simulink model "uniaxial_table"  (R2023b)
settings: Solver=ode8  StartTime=0.0  StopTime=30  FixedStep=t_step  MaxStep=1e-6  RelTol=1e-6
values from neighbouring files (symbols this model uses):
  A = 0.012456    [Compute_TFs_and_StateSpace.m]    (also in parameters.m)
  C_l = k_c    (= 8.37005e-08)    [parameters.m]
  c_sp = qsi_sp*2*m_sp*2*pi*f_sp    (= 2513.27412287)    [parameters.m]
  c_t = 5.7800    (= 5.78)    [parameters.m]
  k_c = k_pl/2    (= 8.37005e-08)    [parameters.m]
  K_h = 4*beta_e*A^2/V_t    (= 45213.1716837)    [parameters.m]
  k_p = 1.2993/1e-2    (= 129.93)    [Copy_of_PID_surf_Zeta.m]    (also in PID_surface.m; parameters.m = 1.2993)
  k_q = 1934.50    (= 1934.5)    [parameters.m]
  k_sp = m_sp*(2*pi*f_sp)^2    (= 315827.340835)    [parameters.m]
  k_sv = 1934.50    (= 1934.5)    [parameters.m]
  m_sp = 2000    [parameters.m]
  m_T = m_p    (= 1.9751)    [parameters.m]
  tau_sv = 0.0246    [Compute_TFs_and_StateSpace.m]    (also in parameters.m)
libraries: slpidlib x1
settings Model: Creator=afons  LastModifiedBy=afons

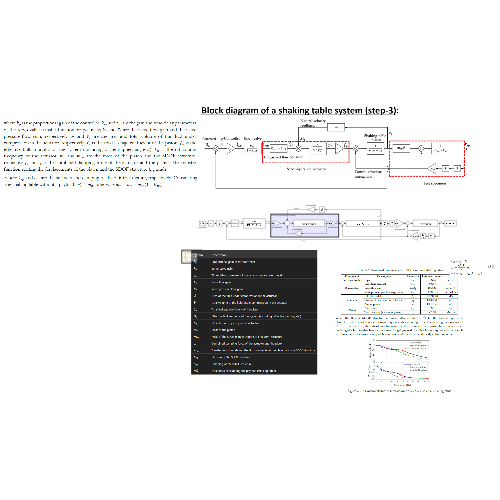
[thumbnail: Simulink's stored preview of the top-level diagram]
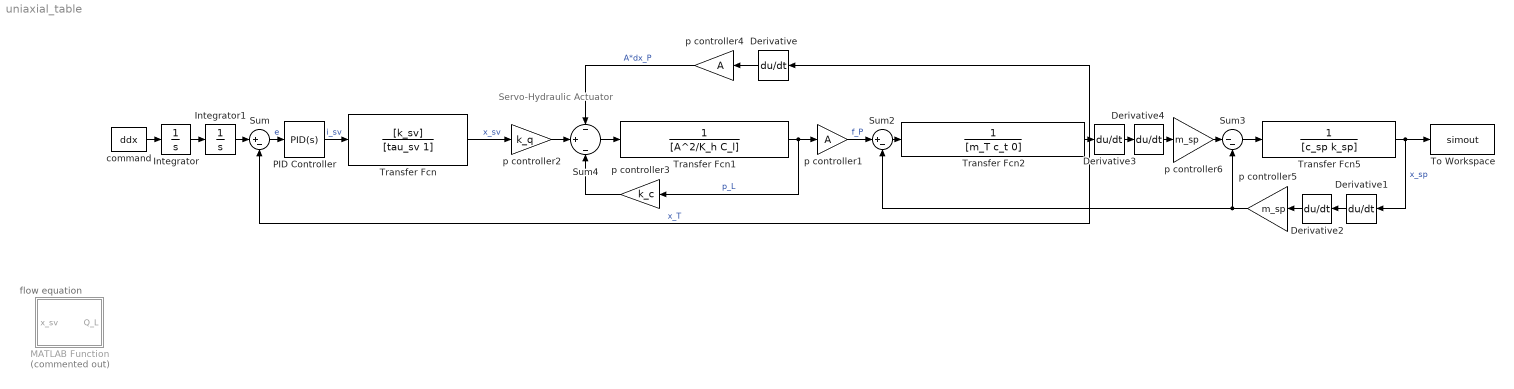
== system uniaxial_table ==
  note: Servo-Hydraulic Actuator
  note: flow equation
  Derivative{,1..4} (5 alike) : Derivative
  Integrator : Integrator
  Integrator1 : Integrator
  MATLAB Function : MATLAB Function  Commented=on  TreatAsAtomicUnit=on
  PID Controller : slpidlib/PID Controller  Controller=PID  Form=Parallel  TimeDomain=Continuous-time  UseExternalTs=off  SampleTime=-1  IntegratorMethod=Forward Euler  FilterMethod=Forward Euler  ControllerParametersSource=internal  P=k_p  I=0  UseKiTs=off  D=0  N=1  UseFilter=on  TunerSelectOption=Transfer Function Based (PID Tuner App)  InitialConditionSource=internal  InitialConditionForIntegrator=0  InitialConditionForFilter=0  DifferentiatorICPrevScaledInput=0  ExternalReset=none  TrackingMode=off  Kt=1  LimitOutput=off  SatLimitsSource=internal  UpperSaturationLimit=inf  LowerSaturationLimit=-inf  LinearizeAsGain=on  AntiWindupMode=none  Kb=1  LimitIntegrator=off  UpperIntegratorSaturationLimit=inf  LowerIntegratorSaturationLimit=-inf  POutMin=[]  POutMax=[]  IOutMin=[]  IOutMax=[]  DOutMin=[]  DOutMax=[]  NOutMin=[]  NOutMax=[]  SumOutMin=[]  SumOutMax=[]  SaturationOutMin=[]  SaturationOutMax=[]  PParamMin=[]  PParamMax=[]  IParamMin=[]  IParamMax=[]  DParamMin=[]  DParamMax=[]  NParamMin=[]  NParamMax=[]  KbParamMin=[]  KbParamMax=[]  KtParamMin=[]  KtParamMax=[]  KbOutMin=[]  KbOutMax=[]  KtOutMin=[]  KtOutMax=[]  IntegratorOutMin=[]  IntegratorOutMax=[]  FilterOutMin=[]  FilterOutMax=[]  SumI1OutMin=[]  SumI1OutMax=[]  SumI2OutMin=[]  SumI2OutMax=[]  SumI3OutMin=[]  SumI3OutMax=[]  SumI4OutMin=[]  SumI4OutMax=[]  SumDOutMin=[]  SumDOutMax=[]  DifferentiatorOutMin=[]  DifferentiatorOutMax=[]  FilterDiffOutCoefMin=[]  FilterDiffOutCoefMax=[]  ReciprocalOutMin=[]  ReciprocalOutMax=[]  SumDenOutMin=[]  SumDenOutMax=[]  SumNumOutMin=[]  SumNumOutMax=[]  DivideOutMin=[]  DivideOutMax=[]  UdiffTsProdOutMin=[]  UdiffTsProdOutMax=[]  NTsProdOutMin=[]  NTsProdOutMax=[]  UintegralTsProdOutMin=[]  UintegralTsProdOutMax=[]  UngainTsProdOutMin=[]  UngainTsProdOutMax=[]  ClampingZeroOutDataTypeStr=Inherit: Inherit via back propagation  ClampingZeroOutMin=[]  ClampingZeroOutMax=[]  FilterDenConstantOutDataTypeStr=Inherit: Inherit via back propagation  FilterDenConstantOutMin=[]  FilterDenConstantOutMax=[]  PCopyOutDataTypeStr=Inherit: Inherit via back propagation  PCopyOutMin=[]  PCopyOutMax=[]  NCopyOutDataTypeStr=Inherit: Inherit via back propagation  NCopyOutMin=[]  NCopyOutMax=[]  IntegratorContinuousStateAttributes=''  IntegratorStateMustResolveToSignalObject=off  IntegratorRTWStateStorageClass=Auto  FilterContinuousStateAttributes=''  FilterStateMustResolveToSignalObject=off  FilterRTWStateStorageClass=Auto  ParallelPVariant=InternalParameters  IdealPVariant=Disabled  IVariant=InternalParameters  DVariant=InternalParameters  IntegratorVariant=Continuous  SatVariant=Disabled  AWVariant=Passthrough  PCopyVariant=Disabled  TRVariant=Disabled  FdbkBlocksVariant=Forward  IdealPFdbkVariant=Disabled  SatFdbkVariant=Disabled  DerivativeFilterVariant=ContFilter  NVariant=InternalParameters  NCopyVariant=Disabled  FilterICVariant=InternalICsFilter  IntegratorICVariant=InternalICs  ExternalResetVariant=Disabled  TRSumVariant=Passthrough  SumFdbkVariant=Disabled  SumVariant=Sum_PID  TsampFilterVariant=InternalTs  TsampNgainVariant=Passthrough  TsampIntegralVariant=Disabled_SignalSpec  ExternalSaturationOutDataTypeStr=Inherit: Same as second input
  Sum : Sum  Inputs=|+-
  Sum2 : Sum  Inputs=|+-
  Sum3 : Sum  Inputs=|--
  Sum4 : Sum  Inputs=-|+|-
  To Workspace : ToWorkspace  VariableName=simout  SaveFormat=Timeseries  SampleTime=-1
  Transfer Fcn : TransferFcn  Numerator=[k_sv]  Denominator=[tau_sv 1]
  Transfer Fcn1 : TransferFcn  Denominator=[A^2/K_h C_l]
  Transfer Fcn2 : TransferFcn  Denominator=[m_T c_t 0]
  Transfer Fcn5 : TransferFcn  Denominator=[c_sp k_sp]
  command : FromWorkspace  VariableName=ddx
  p controller1 : Gain  Gain=A
  p controller2 : Gain  Gain=k_q
  p controller3 : Gain  Gain=k_c
  p controller4 : Gain  Gain=A
  p controller5 : Gain  Gain=m_sp
  p controller6 : Gain  Gain=m_sp
  wires:
  Sum/1 -> PID Controller/1  "e"
  PID Controller/1 -> Transfer Fcn/1  "i_sv"
  Transfer Fcn/1 -> p controller2/1  "x_sv"
  Sum4/1 -> Transfer Fcn1/1
  p controller4/1 -> Sum4/1  "A*dx_P"
  Transfer Fcn1/1 -> p controller1/1, p controller3/1  "p_L"
  p controller1/1 -> Sum2/1  "f_P"
  Sum2/1 -> Transfer Fcn2/1
  Transfer Fcn2/1 -> Sum/2, Derivative/1, Derivative3/1  "x_T"
  p controller6/1 -> Sum3/1
  Sum3/1 -> Transfer Fcn5/1
  Transfer Fcn5/1 -> To Workspace/1, Derivative1/1  "x_sp"
  p controller5/1 -> Sum2/2, Sum3/2
  p controller2/1 -> Sum4/2
  p controller3/1 -> Sum4/3
  Derivative/1 -> p controller4/1
  Derivative1/1 -> Derivative2/1
  Derivative2/1 -> p controller5/1
  command/1 -> Integrator/1
  Integrator/1 -> Integrator1/1
  Integrator1/1 -> Sum/1
  Derivative4/1 -> p controller6/1
  Derivative3/1 -> Derivative4/1

== matlab function uniaxial_table/MATLAB Function ==
  data: x_sv input; Q_L output
function Q_L = fcn(x_sv)
%#codegen

Q_L = k_q*x_sv - k_c*p_L ;
